simulink model "Method_1_Jerk_Based"  (R2020b)
settings: Solver=VariableStepAuto  StartTime=0.0  StopTime=320  RelTol=1e-3
values from neighbouring files (symbols this model uses):
  GR = 5    [Model_Data.mat]
  m = 220    [Model_Data.mat]
  r = 0.3059    [Model_Data.mat]
  s2_5_rps = [0 104.6666667 209.3333333 314 418.6666667 523.3333333 628]    [Model_Data.mat]
  s2_5_trq = [70 65 60 50 40 33 27]    [Model_Data.mat]
undefined symbols (not defined in the file or in its folder): h, km, s, sigbuilder_block
libraries: autolibshared x4, aerolibconvert2 x2, autolibmappedmotor x1, simulink x1
(part 1 of 3)
settings Model: Creator=User  LastModifiedBy=User

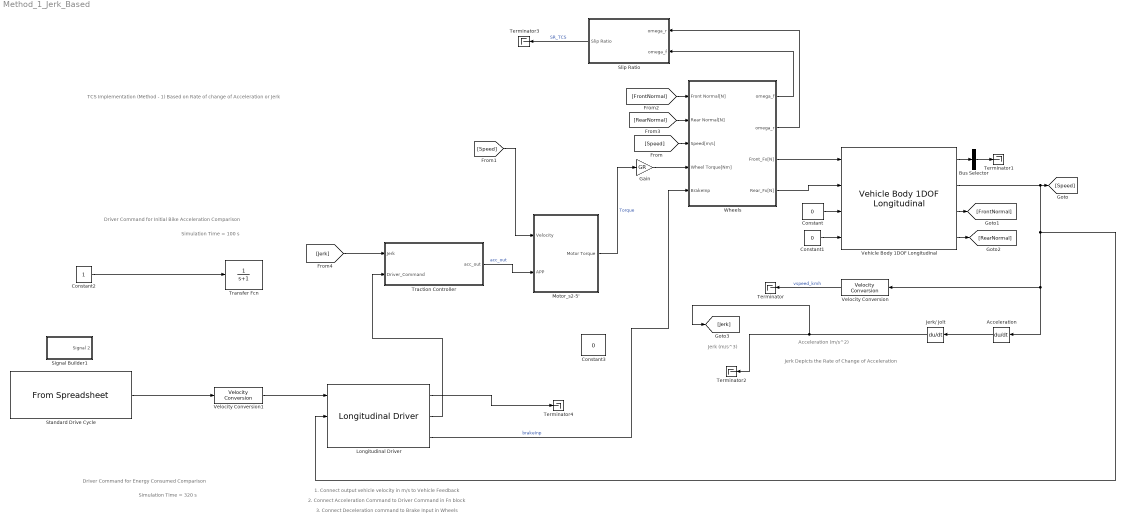
== system Method_1_Jerk_Based ==
  note: Simulation Time = 320 s
  note: Driver Command for Energy Consumed Comparison
  note: 3. Connect Deceleration command to Brake Input in Wheels
  note: 1. Connect output vehicle velocity in m/s to Vehicle Feedback
  note: 2. Connect Acceleration Command to Driver Command in Fn block
  note: Jerk (m/s^3)
  note: Acceleration (m/s^2)
  note: Jerk Depicts the Rate of Change of Acceleration
  note: Driver Command for Initial Bike Acceleration Comparison
  note: Simulation Time = 100 s
  note: TCS Implementation (Method - 1)
      | Based on Rate of change of Acceleration or Jerk
  Acceleration : Derivative
  Bus Selector : BusSelector  OutputSignals=BdyFrm.Cg  OutputAsBus=on
  Constant : Constant  Value=0
  Constant1 : Constant  Value=0
  Constant2 : Constant
  Constant3 : Constant  Value=0
  Gain : Gain  Gain=GR
  Jerk/ Jolt : Derivative
  Longitudinal Driver : autolibshared/Longitudinal Driver  extAccelOvr=off  extDecelOvr=off  extAccelHld=off  extDecelHld=off  extAccelZero=off  extDecelZero=off  cntrlType=PI  shftType=None  velUnits=m/s  gearOut=off  Kp=15  Ki=1  Kff=.05  Kg=.01  VehVelVec=[0 100]  KffVec=[.1 .1]  KpVec=[10 10]  KiVec=[5 5]  KgVec=[0 0]  m=1500  Kpt=3000  tau=.1  L=2  aR=200  bR=2.5  cR=.5  g=9.81  vnom=100  Kaw=.1  tauerr=.03  tauPt=2  GearInit=0  tShift=.1  pdlVec=[0.1 0.4 0.5 0.9]  upShftTbl=[-1 12.9375 26.4375 39.9375 51.18749999999999 62.4375 72.84375 83.25;-1 16.3125 29.8125 43.3125 54.5624 65.8125 76.78125 87.75;-1 19.6875 33.1875 46.68749999999999 57.9375 69.1875 80.71875 92.25;-1 33 52.5 77.25 100.5 138.75 161.875 185]  dwnShftTbl=[1 9.5625 23.0625 36.5625 47.8125 59.0625 68.90625 78.75;1 12.9375 26.4375 39.9375 51.18749999999999 62.4375 72.84375 83.25;1 16.3125 29.8125 43.3125 54.562499 65.8125 76.78125 87.75;1 19.6875 33.1875 46.68749999999999 57.9375 69.1875 80.71875 92.25]  tClutch=.5  tRev=.5  tPark=120  aMode=1  UpGearVec="[0  1  2  3  4  5  6  7]"  DownGearVec="[1  2  3  4  5  6  7  8]"
      settings: SourceProductBaseCode=PW,MT,UV,VE,VP
  "Motor_s2-5' " : Subsystem
  Signal Builder1 : Subsystem  Tag=STV Subsys  LoadFcn=sigbuilder_block('load');  StartFcn=sigbuilder_block('start');  StopFcn=sigbuilder_block('stop');  ClipboardFcn=sigbuilder_block('clipboard');  mask(Sigbuilder block){tuvar=[0:10]}
      mask help: Simulink:masks:SigbuilderBlock_MD
      mask init:
      | if ~strcmp(get_param(bdroot(gcbh),'SimulationStatus'),'stopped') tuvar = sigbuilder_block('maskInit'); end
      settings: CopyFcn=sigbuilder_block('copy');  DeleteFcn=sigbuilder_block('delete');  ModelCloseFcn=sigbuilder_block('modelClose');  PreSaveFcn=sigbuilder_block('preSave');  PauseFcn=sigbuilder_block('pause');  ContinueFcn=sigbuilder_block('continue');  NameChangeFcn=sigbuilder_block('namechange');  OpenFcn=sigbuilder_block('open',[6 30 1012.5 447.75 ]);  CloseFcn=sigbuilder_block('close');
      mask Display: plot(0, 0, 100, 100,[2, 2, 32, 32, 2], [68, 8, 8, 68, 68],[32, 2], [38, 38], [32, 19, 2],[53, 60, 44], [32, 17, 17, 2],[16, 16, 31, 31]);txt = getActiveGroup(gcbh);text(2, 100, txt,'verticalAlignment', 'top');
  Slip Ratio : Subsystem
  Standard Drive Cycle : FromSpreadsheet  FileName=C:\Users\User\Downloads\dc1607 (1).xlsx  SheetName=ehigh
  Terminator{,1..4} (5 alike) : Terminator
  Traction Controller : MATLAB Function  TreatAsAtomicUnit=on
  Transfer Fcn : TransferFcn  Denominator=[1 1]
  Vehicle Body 1DOF Longitudinal : autolibshared/Vehicle Body 1DOF Longitudinal  VariantControl=SL  extFMode=off  extMMode=off  extTamb=off  wind3D=off  aMode=1  NF=1  NR=1  m=m  a=0.736  b=0.706  h=0.597  Cd=Cd  Cl=0  Cpm=0  Af=FrontalArea  x_o=0  xdot_o=0  Pabs=101325  T=273  g=9.81
      settings: SourceProductBaseCode=PW,MT,UV,VE,VP
  Velocity Conversion : aerolibconvert2/Velocity Conversion  IU=m/s  OU=km/h
  Velocity Conversion1 : aerolibconvert2/Velocity Conversion  IU=km/h  OU=m/s
  Wheels : Subsystem
  wires:
  Longitudinal Driver/1 -> Terminator4/1
  Standard Drive Cycle/1 -> Velocity Conversion1/1
  Velocity Conversion1/1 -> Longitudinal Driver/1
  Wheels/1(omega_f) -> Slip Ratio/2(omega_f)
  Bus Selector/1 -> Terminator1/1
  Velocity Conversion/1 -> Terminator/1  "vspeed_kmh"
  Slip Ratio/1(Slip Ratio) -> Terminator3/1  "SR_TCS"
  [Jerk] -> Traction Controller/1(Jerk)
  [FrontNormal] -> Wheels/1(Front Normal[N])
  Constant1/1 -> Vehicle Body 1DOF Longitudinal/4
  Vehicle Body 1DOF Longitudinal/3 -> [FrontNormal]
  [RearNormal] -> Wheels/2(Rear Normal[N])
  Vehicle Body 1DOF Longitudinal/1 -> Bus Selector/1
  Vehicle Body 1DOF Longitudinal/4 -> [RearNormal]
  Acceleration/1 -> Jerk/ Jolt/1
  Wheels/4(Rear_Fx[N]) -> Vehicle Body 1DOF Longitudinal/2
  Constant2/1 -> Transfer Fcn/1
  Wheels/3(Front_Fx[N]) -> Vehicle Body 1DOF Longitudinal/1
  Traction Controller/1(acc_out) -> "Motor_s2-5' "/2(APP)  "acc_out"
  Gain/1 -> Wheels/4(Wheel Torque[Nm])
  [Speed] -> Wheels/3(Speed[m/s])
  "Motor_s2-5' "/1(Motor Torque) -> Gain/1  "Torque"
  Constant/1 -> Vehicle Body 1DOF Longitudinal/3
  Vehicle Body 1DOF Longitudinal/2 -> Acceleration/1, Velocity Conversion/1, Longitudinal Driver/2, [Speed]
  [Speed] -> "Motor_s2-5' "/1(Velocity)
  Jerk/ Jolt/1 -> Terminator2/1, [Jerk]
  Wheels/2(omega_r) -> Slip Ratio/1(omega_r)
  Longitudinal Driver/2 -> Traction Controller/2(Driver_Command)
  Longitudinal Driver/3 -> Wheels/5(BrakeInp)  "brakeInp"

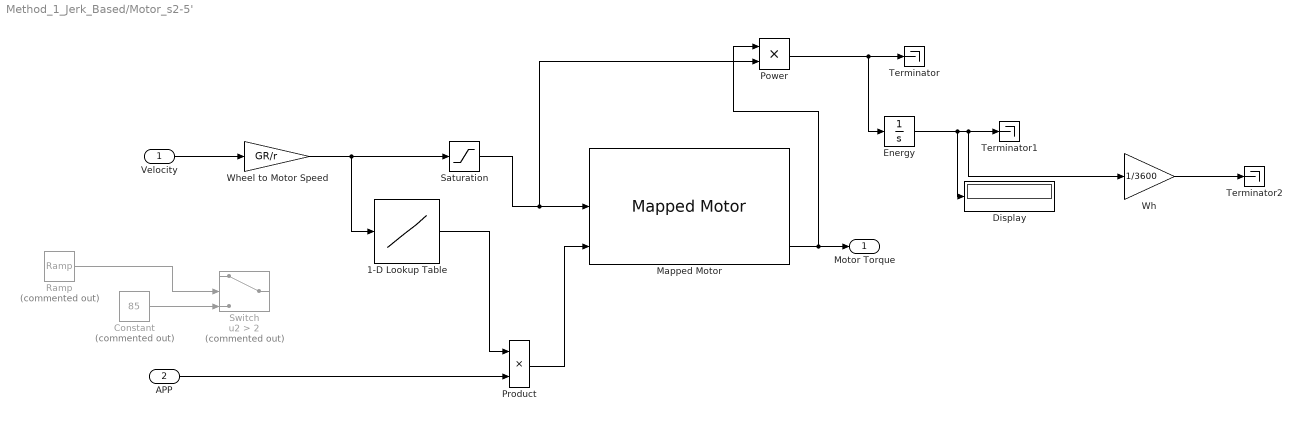
== system Method_1_Jerk_Based/Motor_s2-5'  ==
  Velocity : Inport
  APP : Inport  Port=2
  1-D Lookup Table : Lookup_n-D  NumberOfTableDimensions=1  BreakpointsForDimension1=s2_5_rps  Table=s2_5_trq  InternalRulePriority=Speed  RndMeth=Simplest  InputSameDT=on
  Constant : Constant  Commented=on  Value=85
  Display : Display
  Energy : Integrator
  Mapped Motor : autolibmappedmotor/Mapped Motor  port_config=Speed  param_by=Tabulated torque-speed envelope  w_t=s2_5_rps  T_t=s2_5_trq  torque_max=.1  power_max=30  Tc=0.02  param_loss=Single efficiency measurement  eff=90  w_eff=360  T_eff=29.3  Piron=0  Pbase=0  w_eff_bp=[-8000 -4000 0 4000 8000]  T_eff_bp=[0 0.03 0.06 0.09]  Temp_eff_bp=[233.15 293.15 373.15]  losses_table=[1.49 1.67 2.21 3.10; 0.42 0.69 1.14 2.03; 0.06 0.24 0.78 1.68; 0.42 0.69 1.14 2.03; 1.49 1.67 2.21 3.10]  losses_table_3d=cat(3,1.05*[1.49 1.67 2.21 3.10; 0.42 0.69 1.14 2.03; 0.06 0.24 0.78 1.68; 0.42 0.69 1.14 2.03; 1.49 1.67 2.21 3.10],[1.49 1.67 2.21 3.10; 0.42 0.69 1.14 2.03; 0.06 0.24 0.78 1.68; 0.42 0.69 1.14 2.03; 1.49 1.67 2.21 3.10],1.03*[1.49 1.67 2.21 3.10; 0.42 0.69 1.14 2.03; 0.06 0.24 0.78 1.68; 0.42 0.69 1.14 2.03; 1.49 1.67 2.21 3.10])  efficiency_table=[95 95 95 95; 95 95 95 95; 95 95 95 95; 95 95 95 95; 95 95 95 95]  efficiency_table_3d=cat(3,90*ones(5,4),95*ones(5,4),92*ones(5,4))  J=5e-6  b=1e-5  omega_o=0  T_t_extended=[27 33 40 50 60 65 70 65 60 50 40 33 27]  w_t_extended=[-628 -523.3333333 -418.6666667 -314 -209.3333333 -104.6666667 0 104.6666667 209.3333333 314 418.6666667 523.3333333 628]  KLossIron=0  KLossCopper=1.3652  x_w_eff_vec=[-8000 -4000 0 4000 8000]  x_T_eff_vec=[-0.09 -0.06 -0.03 0 0.03 0.06 0.09]  x_tmp_eff_vec=[233.15 293.15 373.15]  x_losses_mat=[3.1 2.21 1.67 1.49 1.67 2.21 3.1;2.03 1.14 0.69 0.42 0.69 1.14 2.03;1.68 0.78 0.24 0.06 0.24 0.78 1.68;2.03 1.14 0.69 0.42 0.69 1.14 2.03;3.1 2.21 1.67 1.49 1.67 2.21 3.1]  x_losses_mat_3d=cat(3,[3.255 2.3205 1.7535 1.5645 1.7535 2.3205 3.255;2.1315 1.197 0.7245 0.441 0.7245 1.197 2.1315;1.764 0.819 0.252 0.063 0.252 0.819 1.764;2.1315 1.197 0.7245 0.441 0.7245 1.197 2.1315;3.255 2.3205 1.7535 1.5645 1.7535 2.3205 3.255],[3.1 2.21 1.67 1.49 1.67 2.21 3.1;2.03 1.14 0.69 0.42 0.69 1.14 2.03;1.68 0.78 0.24 0.06 0.24 0.78 1.68;2.03 1.14 0.69 0.42 0.69 1.14 2.03;3.1 2.21 1.67 1.49 1.67 2.21 3.1],[3.193 2.2763 1.7201 1.5347 1.7201 2.2763 3.193;2.0909 1.1742 0.7107 0.4326 0.7107 1.1742 2.0909;1.7304 0.8034 0.2472 0.0618 0.2472 0.8034 1.7304;2.0909 1.1742 0.7107 0.4326 0.7107 1.1742 2.0909;3.193 2.2763 1.7201 1.5347 1.7201 2.2763 3.193])  CalLossMapData={}  CalLossWithTempMapData={}  aMode=2  RefBlkName='autolibmappedmotor/Mapped Motor'
      settings: SourceProductBaseCode=PW,MT,UV,VE,VP
  Power : Product
  Product : Product
  Ramp : simulink/Sources/Ramp  Commented=on  slope=1  start=0  InitialOutput=0
  Saturation : Saturate  UpperLimit=800  LowerLimit=0
  Switch : Switch  Commented=on  Criteria=u2 > Threshold  Threshold=2
  Terminator : Terminator
  Terminator1 : Terminator
  Terminator2 : Terminator
  Wh : Gain  Gain=1/3600
  Wheel to Motor Speed : Gain  Gain=GR/r
  Motor Torque : Outport
  wires:
  Wheel to Motor Speed/1 -> Saturation/1, 1-D Lookup Table/1
  Product/1 -> Mapped Motor/3
  Velocity/1 -> Wheel to Motor Speed/1
  Saturation/1 -> Power/2, Mapped Motor/2
  Mapped Motor/3 -> Power/1, Motor Torque/1
  APP/1 -> Product/2
  Ramp/1 -> Switch/2
  Constant/1 -> Switch/3
  1-D Lookup Table/1 -> Product/1
  Power/1 -> Energy/1, Terminator/1
  Energy/1 -> Display/1, Wh/1, Terminator1/1
  Wh/1 -> Terminator2/1

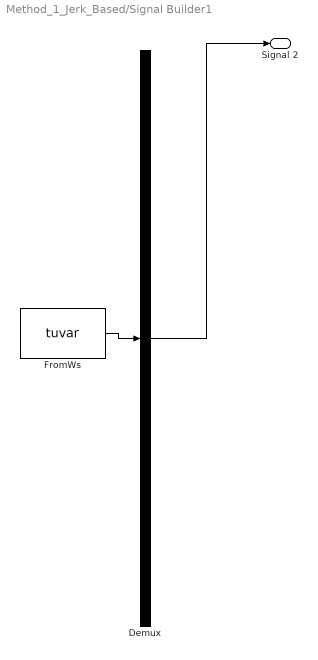
== system Method_1_Jerk_Based/Signal Builder1 ==
  Demux : Demux  Tag=STV Demux  Outputs=1
      settings: DisplayOption=none
  FromWs : FromWorkspace  Tag=STV FromWs  VariableName=tuvar
      SigBuilderData=|
      | common.afterFinalStr = 'Extrapolate'
      | common.sampleTime = 0
      | dataSet.timeRange = [0 100]
      | dataSet.name = 'Group 1'
      | sbobj.Groups.Name = 'Group 1'
      | sbobj.Groups.Signals.Name = 'Signal 2'
      | sbobj.Groups.Signals.XData = [0 1.25 1.25 2.5 3.75 5 6.25 7.5 8.75 10 10 11.25 11.25 12.5 13.75 15 16.25 17.5 18.75 20 21.25 21.25 22.5 23.75 25 26.25 27.5 28.75 30 31.25 32.5 33.75 35 36.25 37.5 38.75 40 41.25 41.25 42.5 43.75 45 45 46.25 46.25 47.5 48.75 50 51.25 52.5 53.75 53.75 55 55 56.25 57.5 58.75 60 61.25 62.5 63.75 65 66.25 67.5 68.75 70 71.25 72.5 73.75 75 76.25 77.5 78.75 80 81.25 82.5 83.75 85 86.25 87.5 88.75 90 91.25 92.5 93.75 95 96.25 97.5 98.75 100]
      | sbobj.Groups.Signals.YData = [0 0.02 0.03 0.08 0.12 0.18 0.2 0.24 0.28 0.32 0.33 0.37 0.42 0.47 0.5 0.54 0.57 0.6 0.61 0.64 0.61 0.625 0.615 0.565 0.515 0.475 0.405 0.315 0.255 0.215 0.175 0.155 0.135 0.095 0.055 0.06 0.04 0.035 0.01 0.025 0.04 0.03 0.055 0.025 0.015 0.015 0 0.035 0.045 0.05 0.01 0.015 0 0.02 0.005 0 0.015 0.05 0 -0.005 -0.005 -0.01 0 0 -0.01 0.055 0.065 0.06 0.08 0.09 0.09 0.09 0.09 0.105 0.14 0.15 0.165 0.175 0.19 0.215 0.292893218813 0.49 0.7 0.76 0.9 0.96 0.292893218813 0 -0.02 0.015]
      | sbobj.Groups.TimeRange = [0 100]
  Signal 2 : Outport  Tag=STV Outport
  wires:
  FromWs/1 -> Demux/1
  Demux/1 -> Signal 2/1

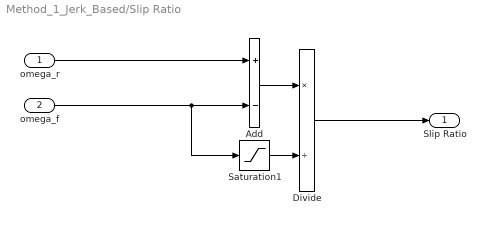
== system Method_1_Jerk_Based/Slip Ratio ==
  omega_r : Inport
  omega_f : Inport  Port=2
  Add : Sum  Inputs=+-
  Divide : Product  Inputs=*/
  Saturation1 : Saturate  UpperLimit=1000  LowerLimit=0.01
  Slip Ratio : Outport  VectorParamsAs1DForOutWhenUnconnected=off
  wires:
  Add/1 -> Divide/1
  Saturation1/1 -> Divide/2
  Divide/1 -> Slip Ratio/1
  omega_f/1 -> Saturation1/1, Add/2
  omega_r/1 -> Add/1
